simulink model "PressureShield_LQ"  (R2019a)
settings: Solver=FixedStepDiscrete  StartTime=0.0  StopTime=55  FixedStep=0.001  RelTol=1e-3  EnableMultiTasking=on
undefined symbols (not defined in the file): Discrete, Time
libraries: ctrlSharedLib x1, PressureLibrary x1, simulink x1
settings Model: ExtModeTrigDuration=2  Creator=staronm3  LastModifiedBy=Gergely
settings SolverCC: AutoInsertRateTranBlk=on
settings OptimizationCC: EnhancedBackFolding=on  PassReuseOutputArgsThreshold=0  MaxStackSize=64  OptimizeBlockOrder=speed  DifferentSizesBufferReuse=on  OptimizationCustomize=off
settings DebuggingCC: ParameterTunabilityLossMsg=error
settings HardwareCC: ProdBitPerInt=16  ProdBitPerPointer=16  ProdBitPerSizeT=16  ProdBitPerPtrDiffT=16  ProdLargestAtomicFloat=None  ProdWordSize=8  ProdHWDeviceType=Atmel->AVR  UseEmbeddedCoderFeatures=off
settings SFSimCC: MATLABDynamicMemAlloc=off
settings RTWCC: SystemTargetFile=ert.tlc  HardwareBoard=Arduino Mega 2560  TLCOptions=-aInlineSetEventsForThisBaseRateFcn=TLC_FALSE -aSuppressMultiTaskScheduler=TLC_FALSE -aRateBasedStepFcn=1  TemplateMakefile=ert_default_tmf  GenerateReport=on  Toolchain=Arduino AVR  BuildConfiguration=Faster Runs  LaunchReport=on
settings CodeAppCC: ForceParamTrailComments=on  OperatorAnnotations=on
settings ERTTargetCC: ERTCustomFileBanners=off  SupportContinuousTime=on  SupportNonInlinedSFcns=on  RemoveResetFunc=off  SupportVariableSizeSignals=on  ModelStepFunctionPrototypeControlCompliant=off  ExtModeStaticAllocSize=2048

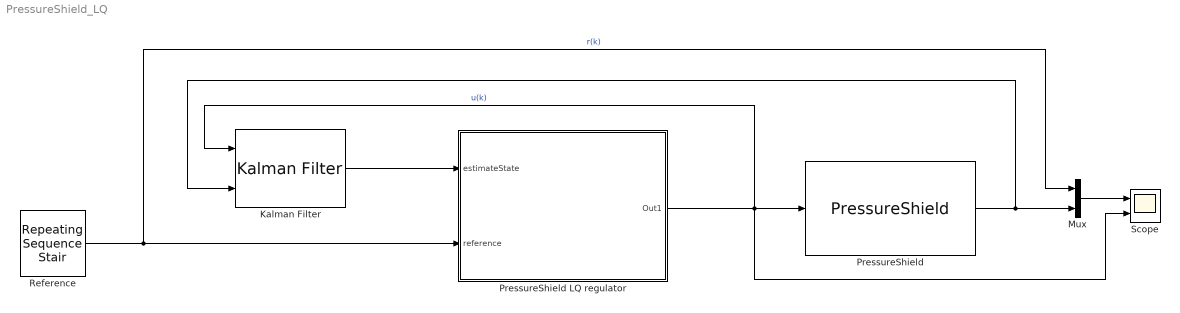
== system PressureShield_LQ ==
  Kalman Filter : ctrlSharedLib/Kalman Filter  TimeDomain=Discrete-Time  UseCurrentEstimator=on  ModelSource=Individual A, B, C, D matrices  ModelSourceVariable=ss(0.95,1,1,0,1)  A=[0.993, 0.01526; -0.003223, 0.4206]  B=[0.008751; -0.1501]  C=[1.74, 0.8755]  D=0  NumberOfStates=1  NumberOfInputs=1  NumberOfOutputs=1  InitialEstimateSource=Dialog  X0=[0;0]  P0=10  UseK=off  UseGH=off  NumberOfProcessNoiseInputs=1  G=1  TimeInvariantG=on  H=0  TimeInvariantH=on  Q=[0.05, 0; 0, 0.01]  TimeInvariantQ=on  R=1  TimeInvariantR=on  N=0  TimeInvariantN=on  AddInputPort=on  AddEnablePort=off  OutputEstimatedY=off  OutputP=off  Ts=0.01
  Mux : Mux  Inputs=2
  "PressureShield " : PressureLibrary/PressureShield    SystemSampleTime=-1  Latency=0  AutoFrameSizeCalculation=off
      link override "Sensor Read/BMP280 ": Ts=0.01
      link override Sensor Read/If Action Subsystem: Ts=0.01
  PressureShield LQ regulator : Subsystem  mask{K=[1.25, 0.05, -0.01], Ts=0.01}
      mask prompts: K "LQ gain"; Ts "Sampling period (s)"
  Reference : simulink/Sources/Repeating Sequence Stair  OutValues=[50 70 40 60 80 60 30 70 60].'  tsamp=5  OutMin=[]  OutMax=[]  OutDataTypeStr=double  OutputDataTypeScalingMode=double  OutDataType=fixdt(0,8)  ConRadixGroup=Best Precision: Vector-wise  OutScaling=2^-12
  Scope : Scope  NumInputPorts=2
  wires:
  PressureShield LQ regulator/1(Out1) -> Kalman Filter/1, "PressureShield "/1, Scope/2  "u(k)"
  Kalman Filter/1 -> PressureShield LQ regulator/1(estimateState)
  Reference/1 -> PressureShield LQ regulator/2(reference), Mux/1  "r(k)"
  Mux/1 -> Scope/1
  "PressureShield "/1 -> Kalman Filter/2, Mux/2

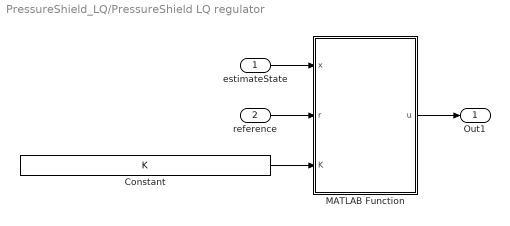
== system PressureShield_LQ/PressureShield LQ regulator ==
  estimateState : Inport
  reference : Inport  Port=2
  Constant : Constant  Value=K  VectorParams1D=off  SampleTime=Ts
  MATLAB Function : MATLAB Function  TreatAsAtomicUnit=on  SystemSampleTime=Ts
  Out1 : Outport
  wires:
  MATLAB Function/1(u) -> Out1/1
  reference/1 -> MATLAB Function/2(r)
  estimateState/1 -> MATLAB Function/1(x)
  Constant/1 -> MATLAB Function/3(K)

== matlab function PressureShield_LQ/PressureShield LQ regulator/MATLAB Function ==
  data: x input; u output; r input; K input
function u = fcn(x, r, K)
persistent xI;
if isempty(xI)    
    xI = 0;
end
xI = xI + r - x(1) - r*0.35;
x = [x; xI];
u = -K * (x - [r;0;0]);
